simulink model "manual_model_features"  (R2020b)
settings: Solver=VariableStepAuto  StartTime=0.0  StopTime=10.0  RelTol=1e-3
undefined symbols (not defined in the file): sigbuilder_block
libraries: simulink x141
(part 1 of 3)
settings Model: Creator=99003757  LastModifiedBy=99003732
settings SFSimCC: CustomCodeUndefinedFunction=UseInterfaceOnly

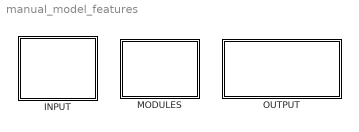
== system manual_model_features ==
  INPUT : Subsystem
  MODULES : Subsystem
  OUTPUT : Subsystem

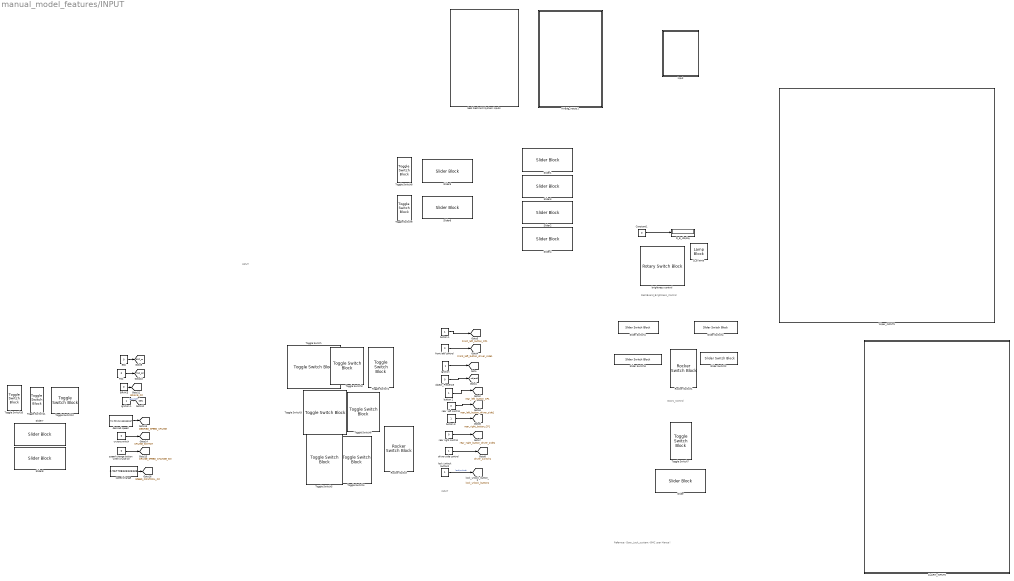
== system manual_model_features/INPUT ==
  note: INPUT
  note: INPUT
  note: DashBoard_Brightness_Control
  note: Doors_Control
  note: Refernce:-
      | Door_Lock_system:-GMC user Manua l
  ALARM_INPUTS : Subsystem
  AirBag_Inputs1 : Subsystem
  BRAKE : Constant  Value=0
  Constant1 : Constant  Value=0
  D_B lamp : LampBlock
  D_B_display : Display
  ESC : Constant  Value=0
  Input : Subsystem
  Rocker Switch : RockerSwitchBlock  LabelPosition=Bottom
      settings: Values={{'Off', 'On'}, [0 1]}
  Rocker Switch1 : RockerSwitchBlock
      settings: Values={{'Off', 'On'}, [1 0]}
  Seat Restraint System Inputs : Subsystem
  Slider{,1..8} (9 alike) : SliderBlock
  Slider Switch{1..4} (4 alike) : SliderSwitchBlock
      settings: Values={{'unlock', 'lock'}, [0 1]}
  TSC : Constant  Value=0
  Toggle Switch{,1..12} (13 alike) : ToggleSwitchBlock
  Wiper_INPUTS : Subsystem
  brightness control : RotarySwitchBlock
      settings: Values={{'Off', 'very Low', 'Low', 'medium', 'high', 'very high'}, [0 1 2 3 4 5]}
  "button 1 " : Constant
  button 2 : Constant
  button 3 : Constant
  cruise switch : Constant  Value=0
  desired speed : Constant  Value=51.90104166666667
  driver side control : Constant
  front left control : Constant  Value=0
  "ignition " : Constant
  ignition 1 : Constant
  lock /unlock button2 : Constant
  object_Presence : Constant  Value=0
  rear  left control : Constant  Value=0
  rear right control : Constant  Value=0
  speed change : Constant  Value=3.567708333333333
  "speed change button when cruise on " : Constant  Value=0
  tag scope: BRAKE_CC=global, CRUISE_SPEED_CHANGE_SW=global, CRUISE_SWITCH=global, DESIRED_SPEED_CRUISE=global, ESC_cc=global, Front_left_button_CP1=global, Front_left_button_driver_side1=global, IGN=global, SPEED_CONTROL_CC=global, TSC_CC=global, driver_switch1=global, ignition1=global, lock_unlock_button1=global, object1=global, rear_left_button_CP1=global, rear_left_button_driver_side1=global, rear_right_button_CP1=global, rear_right_button_driver_side1=global
  wires:
  object_Presence/1 -> [object1]
  driver side control/1 -> [driver_switch1]
  Constant1/1 -> D_B_display/1
  button 3/1 -> [rear_right_button_CP1]
  rear right control/1 -> [rear_right_button_driver_side1]
  "ignition "/1 -> [ignition1]
  rear  left control/1 -> [rear_left_button_driver_side1]
  lock /unlock button2/1 -> [lock_unlock_button1]  "lock/unlock"
  button 2/1 -> [rear_left_button_CP1]
  front left control/1 -> [Front_left_button_driver_side1]
  "button 1 "/1 -> [Front_left_button_CP1]
  speed change/1 -> [SPEED_CONTROL_CC]
  desired speed/1 -> [DESIRED_SPEED_CRUISE]
  ESC/1 -> [ESC_cc]
  ignition 1/1 -> [IGN]  "igswitch"
  "speed change button when cruise on "/1 -> [CRUISE_SPEED_CHANGE_SW]
  BRAKE/1 -> [BRAKE_CC]
  TSC/1 -> [TSC_CC]
  cruise switch/1 -> [CRUISE_SWITCH]

== system manual_model_features/MODULES ==
  "\tPOWER_WINDOW" : Subsystem
  ALARM_SYSTEM : Subsystem
  AirBagSystem : Subsystem
  AirBagSystem2 : Subsystem
  CRUISE_CONTROL : Subsystem
  Door_System : Subsystem
  SeatRestraintSystem1 : Subsystem
  Subsystem2 : Subsystem
  Tire Pressure Monitoring System : Subsystem
  WIPER_CONTROL : Subsystem
  system : Subsystem

== system manual_model_features/OUTPUT ==
  note: Roof light
  note: Signal status
  note: roof light
  ALARM_OUTPUT1 : Subsystem
  Air_Bag_Output : Subsystem
  Cruise_output : Subsystem
  Lamp : LampBlock
  OUTPUT : Subsystem
  OUTPUT1 : Subsystem
  OUTPUT2 : Subsystem
  Output : Subsystem
  Outputs1 : Subsystem
  TP1_Indicator : LampBlock
  TP2_Indicator : LampBlock
  TP3_Indicator : LampBlock
  TP4_Indicator : LampBlock
  automatic door lamp status : LampBlock
  delay lamp status : LampBlock

== system manual_model_features/INPUT/ALARM_INPUTS ==
  Signal Builder : Subsystem  Tag=STV Subsys  LoadFcn=sigbuilder_block('load');  StartFcn=sigbuilder_block('start');  StopFcn=sigbuilder_block('stop');  ClipboardFcn=sigbuilder_block('clipboard');  mask(Sigbuilder block){tuvar=[0:10]}
      mask help: Simulink:masks:SigbuilderBlock_MD
      mask init:
      | if ~strcmp(get_param(bdroot(gcbh),'SimulationStatus'),'stopped') tuvar = sigbuilder_block('maskInit'); end
      settings: CopyFcn=sigbuilder_block('copy');  DeleteFcn=sigbuilder_block('delete');  ModelCloseFcn=sigbuilder_block('modelClose');  PreSaveFcn=sigbuilder_block('preSave');  PauseFcn=sigbuilder_block('pause');  ContinueFcn=sigbuilder_block('continue');  NameChangeFcn=sigbuilder_block('namechange');  OpenFcn=sigbuilder_block('open',[403.5 199.2 550.5 359.55 ]);  CloseFcn=sigbuilder_block('close');
      mask Display: plot(0, 0, 100, 100,[2, 2, 32, 32, 2], [68, 8, 8, 68, 68],[32, 2], [38, 38], [32, 19, 2],[53, 60, 44], [32, 17, 17, 2],[16, 16, 31, 31]);txt = getActiveGroup(gcbh);text(2, 100, txt,'verticalAlignment', 'top');
  tag scope: AS_Doors=global, CAR_ON=global, Ignition=global, RKE=global
  wires:
  Signal Builder/1(AS_Doors) -> [AS_Doors]
  Signal Builder/2(Ignition) -> [Ignition]
  Signal Builder/3(Car_ON) -> [CAR_ON]
  Signal Builder/4(RKE) -> [RKE]

== system manual_model_features/INPUT/AirBag_Inputs1 ==
  Vehicle_Speed : RotarySwitchBlock
      settings: Values={{'50kmph', '80kmph', '100kmph', '140kmph', '180kmph', '230kmph'}, [50 80 100 140 180 230]}
  YawRateMeasure : RotarySwitchBlock
      settings: Values={{'Forward', 'Turning'}, [50 100]}

== system manual_model_features/INPUT/Input ==
  Signal Builder1 : Subsystem  Tag=STV Subsys  LoadFcn=sigbuilder_block('load');  StartFcn=sigbuilder_block('start');  StopFcn=sigbuilder_block('stop');  ClipboardFcn=sigbuilder_block('clipboard');  mask(Sigbuilder block){tuvar=[0:10]}
      mask help: Simulink:masks:SigbuilderBlock_MD
      mask init:
      | if ~strcmp(get_param(bdroot(gcbh),'SimulationStatus'),'stopped') tuvar = sigbuilder_block('maskInit'); end
      settings: CopyFcn=sigbuilder_block('copy');  DeleteFcn=sigbuilder_block('delete');  ModelCloseFcn=sigbuilder_block('modelClose');  PreSaveFcn=sigbuilder_block('preSave');  PauseFcn=sigbuilder_block('pause');  ContinueFcn=sigbuilder_block('continue');  NameChangeFcn=sigbuilder_block('namechange');  OpenFcn=sigbuilder_block('open',[6 37.5 329.25 111.75 ]);  CloseFcn=sigbuilder_block('close');
      mask Display: plot(0, 0, 100, 100,[2, 2, 32, 32, 2], [68, 8, 8, 68, 68],[32, 2], [38, 38], [32, 19, 2],[53, 60, 44], [32, 17, 17, 2],[16, 16, 31, 31]);txt = getActiveGroup(gcbh);text(2, 100, txt,'verticalAlignment', 'top');
  tag scope: ADl_Ignition_System=global, D_sys_Door1=global, D_sys_Door2=global, D_sys_Door3=global, D_sys_Door4=global, D_sys_antilock=global, accln=global
  wires:
  Signal Builder1/1(ignition status) -> [ADl_Ignition_System]
  Signal Builder1/2(Door_1) -> [D_sys_Door1]
  Signal Builder1/3(Door_2) -> [D_sys_Door2]
  Signal Builder1/4(Door_3) -> [D_sys_Door3]
  Signal Builder1/5(Door_4) -> [D_sys_Door4]
  Signal Builder1/6(antilockleature) -> [D_sys_antilock]
  Signal Builder1/7(accln) -> [accln]

== system manual_model_features/INPUT/Seat Restraint System Inputs ==
  Rotary Switch : RotarySwitchBlock
      settings: Values={{'RearAdjust', 'SeatAdjust', 'CushionAdjust', 'Lock'}, [0 1 2 3]}
  SliderForCushionAdjust : SliderBlock
  SliderForRearAdjust : SliderBlock
  SliderForSeatAdjust1 : SliderBlock
  Toggle Switch1 : ToggleSwitchBlock
      settings: Values={{'Off', 'On'}, [0 1]}
  Toggle Switch2 : ToggleSwitchBlock
      settings: Values={{'Off', 'On'}, [0 1]}
  Toggle Switch3 : ToggleSwitchBlock
      settings: Values={{'Off', 'On'}, [0 1]}

== system manual_model_features/INPUT/Wiper_INPUTS ==
  Signal Builder : Subsystem  Tag=STV Subsys  LoadFcn=sigbuilder_block('load');  StartFcn=sigbuilder_block('start');  StopFcn=sigbuilder_block('stop');  ClipboardFcn=sigbuilder_block('clipboard');  mask(Sigbuilder block){tuvar=[0:10]}
      mask help: Simulink:masks:SigbuilderBlock_MD
      mask init:
      | if ~strcmp(get_param(bdroot(gcbh),'SimulationStatus'),'stopped') tuvar = sigbuilder_block('maskInit'); end
      settings: CopyFcn=sigbuilder_block('copy');  DeleteFcn=sigbuilder_block('delete');  ModelCloseFcn=sigbuilder_block('modelClose');  PreSaveFcn=sigbuilder_block('preSave');  PauseFcn=sigbuilder_block('pause');  ContinueFcn=sigbuilder_block('continue');  NameChangeFcn=sigbuilder_block('namechange');  OpenFcn=sigbuilder_block('open',[437.6 199.2 550.4 400 ]);  CloseFcn=sigbuilder_block('close');
      mask Display: plot(0, 0, 100, 100,[2, 2, 32, 32, 2], [68, 8, 8, 68, 68],[32, 2], [38, 38], [32, 19, 2],[53, 60, 44], [32, 17, 17, 2],[16, 16, 31, 31]);txt = getActiveGroup(gcbh);text(2, 100, txt,'verticalAlignment', 'top');
  tag scope: FC_ManualInput=global, FW_Modes=global, WC_BackS=global, WC_FrontS=global, WC_Status=global
  wires:
  Signal Builder/1(FC_Modes) -> [FW_Modes]
  Signal Builder/2(FC_ManualInput) -> [FC_ManualInput]
  Signal Builder/3(WC_BackS) -> [WC_BackS]
  Signal Builder/4(WC_Fronts) -> [WC_FrontS]
  Signal Builder/5(WC_Status) -> [WC_Status]

== system manual_model_features/MODULES/	POWER_WINDOW ==
  Subsystem4 : Subsystem
  tag scope: FL_out=global, FL_warn=global, RL_out=global, RL_warn=global, RR_out=global, RR_warn=global, driver_side_output=global, driver_warn=global
  wires:
  Subsystem4/2(Out_FL) -> [FL_out]
  Subsystem4/1(Out_warn) -> [FL_warn]
  Subsystem4/4(Out_RL) -> [RL_out]
  Subsystem4/6(Out_RR) -> [RR_out]
  [object1] -> Subsystem4/2(object)
  [ignition1] -> Subsystem4/1(Ig_sw)
  Subsystem4/3(Out_RL_warn) -> [RL_warn]
  Subsystem4/8(Out_DC) -> [driver_side_output]
  Subsystem4/5(Out_RR_warn) -> [RR_warn]
  Subsystem4/7(Out_DC_warn) -> [driver_warn]

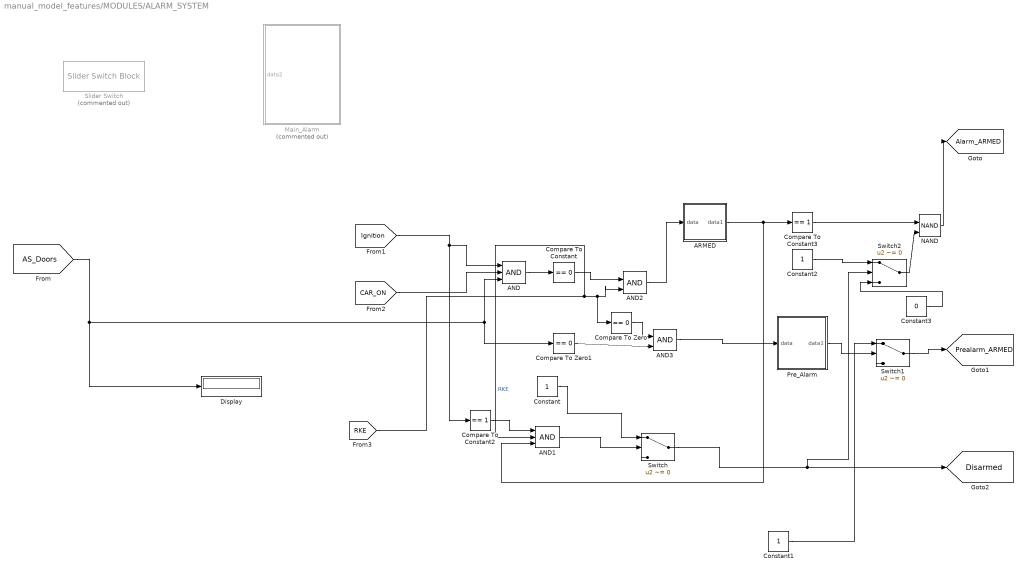
== system manual_model_features/MODULES/ALARM_SYSTEM ==
  AND : Logic  Inputs=3  IconShape=distinctive  AllPortsSameDT=off  OutDataTypeStr=boolean
  AND1 : Logic  Inputs=3  IconShape=distinctive  AllPortsSameDT=off  OutDataTypeStr=boolean
  AND2 : Logic  IconShape=distinctive  AllPortsSameDT=off  OutDataTypeStr=boolean
  AND3 : Logic  IconShape=distinctive  AllPortsSameDT=off  OutDataTypeStr=boolean
  ARMED : Stateflow chart  TreatAsAtomicUnit=on
  Compare To Constant : simulink/Logic and Bit Operations/Compare To Constant  relop===  const=0  OutDataTypeStr=boolean
  Compare To Constant2 : simulink/Logic and Bit Operations/Compare To Constant  relop===  const=1  OutDataTypeStr=boolean
  Compare To Constant3 : simulink/Logic and Bit Operations/Compare To Constant  relop===  const=1  OutDataTypeStr=boolean
  Compare To Zero : simulink/Logic and Bit Operations/Compare To Zero  relop===  OutDataTypeStr=boolean
  Compare To Zero1 : simulink/Logic and Bit Operations/Compare To Zero  relop===  OutDataTypeStr=boolean
  Constant : Constant
  Constant1 : Constant
  Constant2 : Constant
  Constant3 : Constant  Value=0
  Display : Display
  Main_Alarm : Subsystem  Commented=on
  NAND : Logic  Operator=NAND  IconShape=distinctive  AllPortsSameDT=off  OutDataTypeStr=boolean
  Pre_Alarm : Stateflow chart  TreatAsAtomicUnit=on
  Slider Switch : SliderSwitchBlock  Commented=on
      settings: Values={{'Off', 'On'}, [1 0]}
  Switch : Switch  Criteria=u2 ~= 0
  Switch1 : Switch  Criteria=u2 ~= 0
  Switch2 : Switch  Criteria=u2 ~= 0
  tag scope: Alarm_ARMED=global, Disarmed=global, Prealarm_ARMED=global
  wires:
  [RKE] -> AND1/2, Compare To Zero/1, AND2/2  "RKE"
  Constant/1 -> Switch/1
  Constant1/1 -> Switch1/1
  Compare To Zero1/1 -> AND3/2
  Compare To Constant3/1 -> NAND/1
  [CAR_ON] -> AND/2
  Compare To Zero/1 -> AND3/1
  AND2/1 -> ARMED/1(data)
  Pre_Alarm/1(data1) -> Switch1/2
  Compare To Constant/1 -> AND2/1
  AND1/1 -> Switch/2
  [Ignition] -> Compare To Constant2/1, AND/1
  AND/1 -> Compare To Constant/1
  Compare To Constant2/1 -> AND1/1
  Switch/1 -> Switch2/2, [Disarmed]
  Switch1/1 -> [Prealarm_ARMED]
  ARMED/1(data1) -> AND1/3, Compare To Constant3/1
  AND3/1 -> Pre_Alarm/1(data)
  [AS_Doors] -> Display/1, Compare To Zero1/1, AND/3
  Constant2/1 -> Switch2/1
  Switch2/1 -> NAND/2
  NAND/1 -> [Alarm_ARMED]
  Constant3/1 -> Switch2/3

== system manual_model_features/MODULES/AirBagSystem ==
  AND : Logic  IconShape=distinctive  AllPortsSameDT=off  OutDataTypeStr=boolean
  AND1 : Logic  IconShape=distinctive  AllPortsSameDT=off  OutDataTypeStr=boolean
  ActivateAirBagSensor : MATLAB Function  TreatAsAtomicUnit=on
  DetectDeceleration : Subsystem
  FrontAirBagActivation : Subsystem  TreatAsAtomicUnit=on
  Side/Front : Subsystem
  SideAirBagActivation : Subsystem  TreatAsAtomicUnit=on
  wires:
  AND/1 -> FrontAirBagActivation/1(True), FrontAirBagActivation/Enable
  Side/Front/2(In_Front1) -> AND1/1
  ActivateAirBagSensor/1(AirBagSensor) -> AND1/2, AND/2
  Side/Front/1(In_Front) -> AND/1
  AND1/1 -> SideAirBagActivation/1(True), SideAirBagActivation/Enable
  DetectDeceleration/1(Out1) -> ActivateAirBagSensor/1(SuddenDeceleration)

== system manual_model_features/MODULES/AirBagSystem2 ==
  AND : Logic  IconShape=distinctive  AllPortsSameDT=off  OutDataTypeStr=boolean
  AND1 : Logic  IconShape=distinctive  AllPortsSameDT=off  OutDataTypeStr=boolean
  ActivateAirBagSensor : MATLAB Function  TreatAsAtomicUnit=on
  DetectDeceleration : Subsystem
  FrontAirBagActivation : Subsystem  TreatAsAtomicUnit=on
  FrontAirBagActivation1 : Subsystem  TreatAsAtomicUnit=on
  Side/Front : Subsystem
  wires:
  AND/1 -> FrontAirBagActivation/1(True), FrontAirBagActivation/Enable
  AND1/1 -> FrontAirBagActivation1/1(True), FrontAirBagActivation1/Enable
  DetectDeceleration/1(Out1) -> ActivateAirBagSensor/1(SuddenDeceleration)
  ActivateAirBagSensor/1(AirBagSensor) -> AND1/2, AND/2
  Side/Front/2(In_Front1) -> AND1/1
  Side/Front/1(In_Front) -> AND/1

== system manual_model_features/MODULES/CRUISE_CONTROL ==
  note: IGN
  Display : Display
  MATLAB Function : MATLAB Function  TreatAsAtomicUnit=on
  tag scope: output_cruise=global
  wires:
  [DESIRED_SPEED_CRUISE] -> MATLAB Function/5(DESIRED_SPEED_CRUISE)
  [BRAKE_CC] -> MATLAB Function/3(BRAKE_CC)
  [CRUISE_SWITCH] -> MATLAB Function/6(cs)
  [ESC_cc] -> MATLAB Function/1(ESC_CC)
  [SPEED_CONTROL_CC] -> MATLAB Function/8(speedch)
  MATLAB Function/1(y) -> [output_cruise], Display/1  "output"
  [TSC_CC] -> MATLAB Function/2(TSC_CC)
  [IGN] -> MATLAB Function/4(IGN)
  [CRUISE_SPEED_CHANGE_SW] -> MATLAB Function/7(CRUISE_SPEED_CHANGE_SW)

== system manual_model_features/MODULES/Door_System ==
  AND : Logic  IconShape=distinctive  AllPortsSameDT=off  OutDataTypeStr=boolean
  AutomaticDoorLock : Subsystem
  Compare To Constant : simulink/Logic and Bit Operations/Compare To Constant  relop=>  const=0  OutDataTypeStr=boolean
  Display : Display
  Display1 : Display
  OR1 : Logic  Operator=OR  IconShape=distinctive  AllPortsSameDT=off  OutDataTypeStr=boolean
  delay system door lock and interior light subsystem : Subsystem
  wires:
  AutomaticDoorLock/1(Out1) -> AND/1
  AND/1 -> OR1/1, Display/1
  AutomaticDoorLock/2(Out2) -> AND/2
  Compare To Constant/1 -> OR1/2
  OR1/1 -> Display1/1
  delay system door lock and interior light subsystem/1(Out1) -> Compare To Constant/1

== system manual_model_features/MODULES/SeatRestraintSystem1 ==
  Front Seat : Subsystem  TreatAsAtomicUnit=on
  PowerLumbar : Subsystem
  Subsystem : Subsystem
  wires:
  Subsystem/2(Enable_powerSeat_Adj) -> PowerLumbar/1(PowerLumbar)
  Subsystem/1(Enable_FrontSeat_Adj) -> Front Seat/Enable, Front Seat/1(Front_Seat_Adjust)

== system manual_model_features/MODULES/Subsystem2 ==
  CloseValue : Constant  Value=0
  OpenValue : Constant  Value=100
  Subsystem : Subsystem
  Subsystem1 : Subsystem
  enabling system : Subsystem
  tag scope: output1=global, output2=global
  wires:
  enabling system/1(Outport) -> Subsystem1/1(Enable)
  enabling system/2(enableO) -> Subsystem/1(Enable)
  CloseValue/1 -> Subsystem/2(Inport)
  OpenValue/1 -> Subsystem1/2(Inport)
  Subsystem/1(Outport) -> [output2]
  Subsystem1/1(Outport) -> [output1]

== system manual_model_features/MODULES/Tire Pressure Monitoring System ==
  TP_Monitoring : Subsystem
  Tier1State : Display
  Tier2State : Display
  Tier3State : Display
  Tier4State : Display
  tierPressure1 : Constant  Value=87.46448863636364
  tierPressure2 : Constant  Value=75.64630681818181
  tierPressure3 : Constant  Value=78.37357954545455
  tierPressure4 : Constant  Value=86.10085227272727
  wires:
  TP_Monitoring/2(Out2) -> Tier2State/1
  tierPressure4/1 -> TP_Monitoring/4(tierPressure4a), TP_Monitoring/8(tierPressure4b)
  TP_Monitoring/1(Out1) -> Tier1State/1
  tierPressure1/1 -> TP_Monitoring/5(tierPressure1b), TP_Monitoring/1(tierPressure1a)
  tierPressure3/1 -> TP_Monitoring/3(tierPressure3a), TP_Monitoring/7(tierPressure3b)
  TP_Monitoring/3(Out3) -> Tier3State/1
  tierPressure2/1 -> TP_Monitoring/6(tierPressure2b), TP_Monitoring/2(tierPressure2a)
  TP_Monitoring/4(Out4) -> Tier4State/1

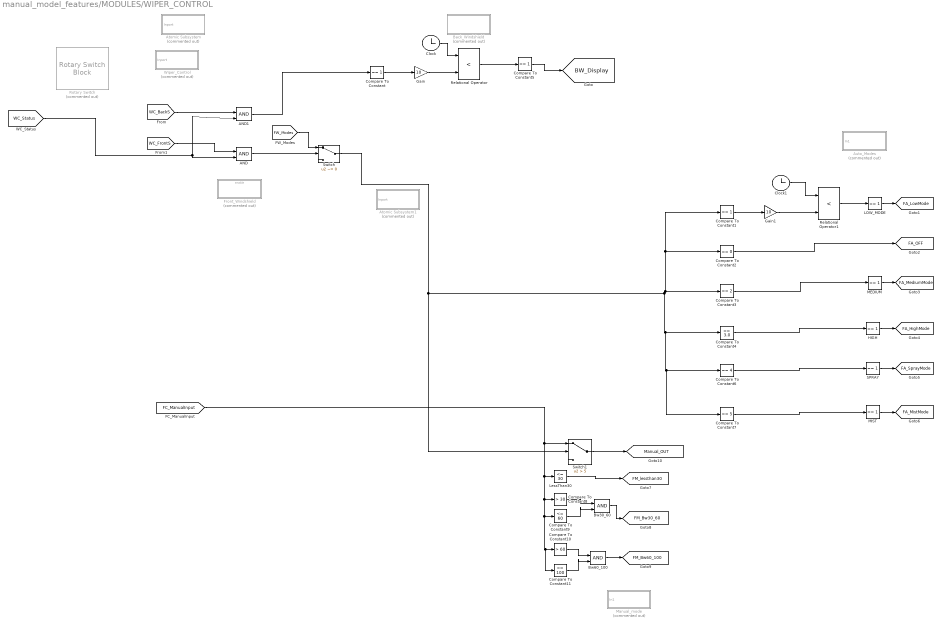
== system manual_model_features/MODULES/WIPER_CONTROL ==
  AND : Logic  IconShape=distinctive  AllPortsSameDT=off  OutDataTypeStr=boolean
  AND1 : Logic  IconShape=distinctive  AllPortsSameDT=off  OutDataTypeStr=boolean
  Atomic Subsystem : Subsystem  Commented=on  TreatAsAtomicUnit=on
  Atomic Subsystem1 : Subsystem  Commented=on  TreatAsAtomicUnit=on
  Auto_Modes : Subsystem  Commented=on
  Back_Windshield : Subsystem  Commented=on  TreatAsAtomicUnit=on
  Bw30_60 : Logic  IconShape=distinctive  AllPortsSameDT=off  OutDataTypeStr=boolean
  Bw60_100 : Logic  IconShape=distinctive  AllPortsSameDT=off  OutDataTypeStr=boolean
  Clock : Clock
      settings: Decimation=5
  Clock1 : Clock
      settings: Decimation=5
  Compare To Constant : simulink/Logic and Bit Operations/Compare To Constant  relop===  const=1  OutDataTypeStr=boolean
  Compare To Constant1 : simulink/Logic and Bit Operations/Compare To Constant  relop===  const=1  OutDataTypeStr=boolean
  Compare To Constant10 : simulink/Logic and Bit Operations/Compare To Constant  relop=>  const=60  OutDataTypeStr=boolean
  Compare To Constant11 : simulink/Logic and Bit Operations/Compare To Constant  relop=<=  const=100  OutDataTypeStr=boolean
  Compare To Constant2 : simulink/Logic and Bit Operations/Compare To Constant  relop===  const=0  OutDataTypeStr=boolean
  Compare To Constant3 : simulink/Logic and Bit Operations/Compare To Constant  relop===  const=2  OutDataTypeStr=boolean
  Compare To Constant4 : simulink/Logic and Bit Operations/Compare To Constant  relop===  const=3.0  OutDataTypeStr=boolean
  Compare To Constant5 : simulink/Logic and Bit Operations/Compare To Constant  relop===  const=1  OutDataTypeStr=boolean
  Compare To Constant6 : simulink/Logic and Bit Operations/Compare To Constant  relop===  const=4  OutDataTypeStr=boolean
  Compare To Constant7 : simulink/Logic and Bit Operations/Compare To Constant  relop===  const=5  OutDataTypeStr=boolean
  Compare To Constant8 : simulink/Logic and Bit Operations/Compare To Constant  relop=>  const=30  OutDataTypeStr=boolean
  Compare To Constant9 : simulink/Logic and Bit Operations/Compare To Constant  relop=<=  const=60  OutDataTypeStr=boolean
  Front_Windshield : Subsystem  Commented=on  TreatAsAtomicUnit=on
  Gain : Gain  Gain=10
  Gain1 : Gain  Gain=10
  HIGH : simulink/Logic and Bit Operations/Compare To Constant  relop===  const=1  OutDataTypeStr=boolean
  LOW_MODE : simulink/Logic and Bit Operations/Compare To Constant  relop===  const=1  OutDataTypeStr=boolean
  LessThan30 : simulink/Logic and Bit Operations/Compare To Constant  relop=<=  const=30  OutDataTypeStr=boolean
  MEDIUM : simulink/Logic and Bit Operations/Compare To Constant  relop===  const=1  OutDataTypeStr=boolean
  MIST : simulink/Logic and Bit Operations/Compare To Constant  relop===  const=1  OutDataTypeStr=boolean
  Manual_mode : Subsystem  Commented=on
  Relational Operator : RelationalOperator  Operator=<  OutDataTypeStr=boolean  RndMeth=Simplest
  Relational Operator1 : RelationalOperator  Operator=<  OutDataTypeStr=boolean  RndMeth=Simplest
  Rotary Switch : RotarySwitchBlock  Commented=on
      settings: Values={{'Off', 'Accessory', 'Ignition'}, [0 1 2]}
  SPRAY : simulink/Logic and Bit Operations/Compare To Constant  relop===  const=1  OutDataTypeStr=boolean
  Switch : Switch  Criteria=u2 ~= 0
  Switch1 : Switch  Criteria=u2 > Threshold  Threshold=5
  Wiper_Control : Subsystem  Commented=on  TreatAsAtomicUnit=on
  tag scope: BW_Display=global, FA_HighMode=global, FA_LowMode=global, FA_MediumMode=global, FA_MistMode=global, FA_OFF=global, FA_SprayMode=global, FM_Bw30_60=global, FM_Bw60_100=global, FM_lessthan30=global, Manual_OUT=global
  wires:
  [WC_Status] -> AND1/2, AND/2
  [WC_BackS] -> AND1/1
  [WC_FrontS] -> AND/1
  Compare To Constant/1 -> Gain/1
  Relational Operator/1 -> Compare To Constant5/1
  Compare To Constant5/1 -> [BW_Display]
  Gain/1 -> Relational Operator/2
  Clock/1 -> Relational Operator/1
  AND1/1 -> Compare To Constant/1
  AND/1 -> Switch/2
  [FW_Modes] -> Switch/1
  Compare To Constant6/1 -> SPRAY/1
  MEDIUM/1 -> [FA_MediumMode]
  HIGH/1 -> [FA_HighMode]
  LOW_MODE/1 -> [FA_LowMode]
  Relational Operator1/1 -> LOW_MODE/1
  Clock1/1 -> Relational Operator1/1
  Gain1/1 -> Relational Operator1/2
  SPRAY/1 -> [FA_SprayMode]
  MIST/1 -> [FA_MistMode]
  Compare To Constant7/1 -> MIST/1
  Compare To Constant2/1 -> [FA_OFF]
  Compare To Constant1/1 -> Gain1/1
  Switch1/1 -> [Manual_OUT]
  [FC_ManualInput] -> Compare To Constant11/1, Compare To Constant10/1, Compare To Constant9/1, Compare To Constant8/1, LessThan30/1, Switch1/1
  Compare To Constant9/1 -> Bw30_60/2
  Switch/1 -> Switch1/2, Compare To Constant7/1, Compare To Constant6/1, Compare To Constant4/1, Compare To Constant3/1, Compare To Constant1/1, Compare To Constant2/1
  LessThan30/1 -> [FM_lessthan30]
  Compare To Constant10/1 -> Bw60_100/1
  Compare To Constant8/1 -> Bw30_60/1
  Compare To Constant11/1 -> Bw60_100/2
  Bw60_100/1 -> [FM_Bw60_100]
  Bw30_60/1 -> [FM_Bw30_60]
  Compare To Constant3/1 -> MEDIUM/1
  Compare To Constant4/1 -> HIGH/1

== system manual_model_features/MODULES/system ==
  note: DOOR LOCK SYSTEM AND INTERIOR LIGHT
  note: Signal status
  note: Doors
  note: Dashboard brightness control
  note: Roof light
  Automatic_Door_lock : Subsystem
  Compare To Constant : simulink/Logic and Bit Operations/Compare To Constant  relop=>  const=0  OutDataTypeStr=boolean
  Constant1 : Constant  Value=0
  Display : Display
  Display1 : Display
  Display2 : Display
  Lamp : LampBlock
  OR1 : Logic  Operator=OR  IconShape=distinctive  AllPortsSameDT=off  OutDataTypeStr=boolean
  Rocker Switch : RockerSwitchBlock
      settings: Values={{'Off', 'On'}, [1 0]}
  Slider : SliderBlock
  Slider Switch{1..4} (4 alike) : SliderSwitchBlock
      settings: Values={{'unlock', 'lock'}, [0 1]}
  Toggle Switch : ToggleSwitchBlock
      settings: Values={{'Off', 'On'}, [0 1]}
  automatic door lamp status : LampBlock
  brightness control : RotarySwitchBlock
      settings: Values={{'Off', 'very Low', 'Low', 'medium', 'high', 'very high'}, [0 1 2 3 4 5]}
  dashboard lamp : LampBlock
  delay lamp status : LampBlock
  delay system door lock and interior light subsystem : Subsystem
  tag scope: A_D_lock=global, D_sys_lock=global
  wires:
  Constant1/1 -> Display2/1
  Compare To Constant/1 -> [D_sys_lock], OR1/2
  delay system door lock and interior light subsystem/1(Out1) -> Compare To Constant/1
  OR1/1 -> Display1/1
  Automatic_Door_lock/1(Out1) -> [A_D_lock], OR1/1, Display/1

== system manual_model_features/OUTPUT/ALARM_OUTPUT1 ==
  note: OUTPUTS
  Display : Display
  Display1 : Display
  Display2 : Display
  Lamp : LampBlock
  wires:
  [Disarmed] -> Display2/1
  [Prealarm_ARMED] -> Display1/1
  [Alarm_ARMED] -> Display/1

== system manual_model_features/OUTPUT/Air_Bag_Output ==
  note: Side Crash (Only the occupied seats are enabled with airbag deployment)
  note: Frontal Crash (Only the occupied seats are enabled with airbag deployment)
  DriverDoorUnlock : LampBlock
  DriverDoorUnlock1 : LampBlock
  DriverFront : LampBlock
  DriverFront1 : LampBlock
  FuelLock{,1..7} (8 alike) : LampBlock
  LeftDoorUnlock : LampBlock
  LeftDoorUnlock1 : LampBlock
  LeftFront : LampBlock
  LeftFront1 : LampBlock
  LeftRear : LampBlock
  LeftRear1 : LampBlock
  LeftRearDoorUnlock : LampBlock
  LeftRearDoorUnlock1 : LampBlock
  RightRear : LampBlock
  RightRear1 : LampBlock
  RightRearDoorUnlock : LampBlock
  RightRearDoorUnlock1 : LampBlock

== system manual_model_features/OUTPUT/Cruise_output ==
  Gauge : CircularGaugeBlock
  Scope : Scope
  wires:
  [output_cruise] -> Scope/1

== system manual_model_features/OUTPUT/OUTPUT ==
  Output_window_scope : Scope  NumInputPorts=4
  Warning_Scope : Scope  NumInputPorts=4
  wires:
  [RR_warn] -> Warning_Scope/3
  [RL_warn] -> Warning_Scope/2
  [FL_warn] -> Warning_Scope/1
  [FL_out] -> Output_window_scope/1
  [RL_out] -> Output_window_scope/2
  [RR_out] -> Output_window_scope/3
  [driver_side_output] -> Output_window_scope/4
  [driver_warn] -> Warning_Scope/4

== system manual_model_features/OUTPUT/OUTPUT1 ==
  Display : Display
  Display1 : Display
  wires:
  [output2] -> Display1/1
  [output1] -> Display/1

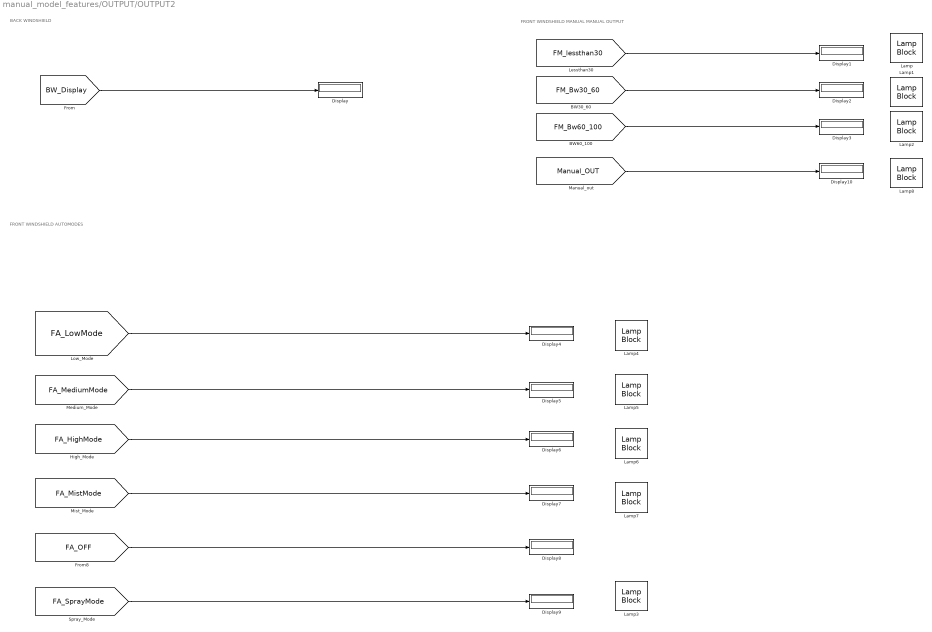
== system manual_model_features/OUTPUT/OUTPUT2 ==
  note: BACK WINDSHIELD
  note: FRONT WINDSHIELD AUTOMODES
  note: FRONT WINDSHIELD MANUAL MANUAL OUTPUT
  Display{,1..10} (11 alike) : Display
  Lamp{,1..8} (9 alike) : LampBlock
  wires:
  [BW_Display] -> Display/1
  [FM_lessthan30] -> Display1/1
  [FM_Bw30_60] -> Display2/1
  [FM_Bw60_100] -> Display3/1
  [FA_LowMode] -> Display4/1
  [FA_MediumMode] -> Display5/1
  [FA_HighMode] -> Display6/1
  [FA_MistMode] -> Display7/1
  [FA_OFF] -> Display8/1
  [FA_SprayMode] -> Display9/1
  [Manual_OUT] -> Display10/1

== system manual_model_features/OUTPUT/Output ==
  Lamp : LampBlock
  Lamp1 : LampBlock
  Lamp2 : LampBlock
  Scope3 : Scope  NumInputPorts=3
  wires:
  [D_Sys_roof] -> Scope3/1
  [A_D_lock] -> Scope3/2
  [D_sys_lock] -> Scope3/3

== system manual_model_features/OUTPUT/Outputs1 ==
  CushionAdjusted : LampBlock
  Front Seat Adjusted : LampBlock
  RearAngleOfSeatAdjust : LampBlock
  SeatUP/DownAdjusted : LampBlock

== system manual_model_features/INPUT/ALARM_INPUTS/Signal Builder ==
  Demux : Demux  Tag=STV Demux
      settings: DisplayOption=none
  FromWs : FromWorkspace  Tag=STV FromWs  VariableName=tuvar
      SigBuilderData=|
      | common.afterFinalStr = 'Extrapolate'
      | common.sampleTime = 0
      | dataSet.timeRange = [0 12]
      | dataSet.name = 'Group 1'
      | sbobj.Groups.Name = 'Group 1'
      | sbobj.Groups.Signals(1).Name = 'AS_Doors'
      | sbobj.Groups.Signals(1).XData = [0 1 2 3 4 5 6 7 8 9 10 11 12]
      | sbobj.Groups.Signals(1).YData = [0 1 1 1 1 1 1 1 1 1 1 1 1]
      | sbobj.Groups.Signals(2).Name = 'Ignition'
      | sbobj.Groups.Signals(2).XData = [0 1 2 3 4 5 6 7 8 9 10 11 12]
      | sbobj.Groups.Signals(2).YData = [0 1 1 1 1 1 1 1 1 1 1 1 1]
      | sbobj.Groups.Signals(3).Name = 'Car_ON'
      | sbobj.Groups.Signals(3).XData = [0 1 2 3 4 5 6 7 8 9 10 11 12]
      | sbobj.Groups.Signals(3).YData = [0 1 1 1 1 1 1 1 1 1 1 1 1]
      | sbobj.Groups.Signals(4).Name = 'RKE'
      | sbobj.Groups.Signals(4).XData = [0 1 2 3 4 5 6 7 8 9 10 11 12]
      | sbobj.Groups.Signals(4).YData = [0 1 1 1 1 1 2 2 2 2 2 2 2]
      | sbobj.Groups.TimeRange = [0 12]
  AS_Doors : Outport  Tag=STV Outport
  Ignition : Outport  Tag=STV Outport  Port=2
  Car_ON : Outport  Tag=STV Outport  Port=3
  RKE : Outport  Tag=STV Outport  Port=4
  wires:
  FromWs/1 -> Demux/1
  Demux/1 -> AS_Doors/1
  Demux/2 -> Ignition/1
  Demux/3 -> Car_ON/1
  Demux/4 -> RKE/1

== system manual_model_features/INPUT/Input/Signal Builder1 ==
  Demux : Demux  Tag=STV Demux  Outputs=7
      settings: DisplayOption=none
  FromWs : FromWorkspace  Tag=STV FromWs  VariableName=tuvar
      SigBuilderData=|
      | common.afterFinalStr = 'Extrapolate'
      | common.sampleTime = 0
      | dataSet.timeRange = [0 30]
      | dataSet.name = 'Group 1'
      | sbobj.Groups.Name = 'Group 1'
      | sbobj.Groups.Signals(1).Name = 'ignition status'
      | sbobj.Groups.Signals(1).XData = [0 1 2 3 4 5 6 7 8 9 10 11 12 13 14 15 16 17 18 19 20 21 22 23 24 25 26 30]
      | sbobj.Groups.Signals(1).YData = [1 1 1 1 1 0 0 0 0 0 0 1 1 1 1 1 1 1 1 1 1 0 0 0 0 0 0 0]
      | sbobj.Groups.Signals(2).Name = 'Door_1'
      | sbobj.Groups.Signals(2).XData = [0 1 2 3 4 5 6 7 8 9 10 11 12 13 14 15 16 17 18 19 20 21 22 23 24 25 26 30]
      | sbobj.Groups.Signals(2).YData = [1 1 1 1 1 1 1 1 1 1 1 1 1 1 1 1 1 1 1 1 1 0 0 0 0 0 0 0]
      | sbobj.Groups.Signals(3).Name = 'Door_2'
      | sbobj.Groups.Signals(3).XData = [0 1 2 3 4 5 6 7 8 9 10 11 12 13 14 15 16 17 18 19 20 21 22 23 24 25 26 30]
      | sbobj.Groups.Signals(3).YData = [1 1 1 1 1 1 1 1 1 1 1 1 1 1 1 1 1 1 1 1 1 0 0 0 0 0 0 0]
      | sbobj.Groups.Signals(4).Name = 'Door_3'
      | sbobj.Groups.Signals(4).XData = [0 1 2 3 4 5 6 7 8 9 10 11 12 13 14 15 16 17 18 19 20 21 22 23 24 25 26 30]
      | sbobj.Groups.Signals(4).YData = [1 1 1 1 1 1 1 1 1 1 1 1 1 1 1 1 1 1 1 1 1 0 0 0 0 0 0 0]
      | sbobj.Groups.Signals(5).Name = 'Door_4'
      | sbobj.Groups.Signals(5).XData = [0 1 2 3 4 5 6 7 8 9 10 11 12 13 14 15 16 17 18 19 20 21 22 23 24 25 26 30]
      | sbobj.Groups.Signals(5).YData = [1 1 1 1 1 1 1 1 1 1 1 1 1 1 1 1 1 1 1 1 1 0 0 0 0 0 0 0]
      | sbobj.Groups.Signals(6).Name = 'antilockleature'
      | sbobj.Groups.Signals(6).XData = [0 1 2 3 4 5 6 7 8 9 10 11 12 13 14 15 16 17 18 19 20 21 22 23 24 25 26 30]
      | sbobj.Groups.Signals(6).YData = [1 1 1 1 1 1 1 1 1 1 1 1 1 1 1 1 1 1 1 1 1 1 1 0 0 0 0 0]
      | sbobj.Groups.Signals(7).Name = 'accln'
      | sbobj.Groups.Signals(7).XData = [0 1 1 2 3 4 5 6 7 8 9 10 11 12 13 14 15 16 17 18 19 20 21 22 23 24 25 26 27 30]
      | sbobj.Groups.Signals(7).YData = [13 14 15 16 17 18 12 20 21 9 10 25 27 29 31 33 35 37 39 41 43 45 47 49 51 53 55 57 59 59]
      | sbobj.Groups.TimeRange = [0 30]
  ignition status : Outport  Tag=STV Outport
  Door_1 : Outport  Tag=STV Outport  Port=2
  Door_2 : Outport  Tag=STV Outport  Port=3
  Door_3 : Outport  Tag=STV Outport  Port=4
  Door_4 : Outport  Tag=STV Outport  Port=5
  antilockleature : Outport  Tag=STV Outport  Port=6
  accln : Outport  Tag=STV Outport  Port=7
  wires:
  FromWs/1 -> Demux/1
  Demux/1 -> ignition status/1
  Demux/2 -> Door_1/1
  Demux/3 -> Door_2/1
  Demux/4 -> Door_3/1
  Demux/5 -> Door_4/1
  Demux/6 -> antilockleature/1
  Demux/7 -> accln/1

== system manual_model_features/INPUT/Wiper_INPUTS/Signal Builder ==
  Demux : Demux  Tag=STV Demux  Outputs=5
      settings: DisplayOption=none
  FromWs : FromWorkspace  Tag=STV FromWs  VariableName=tuvar
      SigBuilderData=|
      | common.afterFinalStr = 'Extrapolate'
      | common.sampleTime = 0
      | dataSet.timeRange = [0 10]
      | dataSet.name = 'Group 1'
      | sbobj.Groups.Name = 'Group 1'
      | sbobj.Groups.Signals(1).Name = 'FC_Modes'
      | sbobj.Groups.Signals(1).XData = [0 1 2 3 4 5 6 7 8 9 10 11 12 13 14 15 16 17 18 19 20 21 22 23 24 25 26 27 28 29 30 31 32 33 34 35 36 37 38 39 40 41 42 43]
      | sbobj.Groups.Signals(1).YData = [0 1 1 1 1 1 1 1 1 1 1 1 2 2 2 2 2 2 2 2 3 3 3 3 3 4 4 4 4 4 5 5 5 6 6 6 6 6 6 6 6 6 6 6]
      | sbobj.Groups.Signals(2).Name = 'FC_ManualInput'
      | sbobj.Groups.Signals(2).XData = [0 1 2 3 4 5 6 7 8 9 10 11 12 13 14 15 16 17 18 19 20 21 22 23 24 25 26 27 28 29 30 31 32 33 34 35 36 37 38 39 40 41 42 43]
      | sbobj.Groups.Signals(2).YData = [0 0 0 0 0 0 0 0 0 0 0 0 0 0 0 0 0 0 0 0 0 0 0 0 0 0 0 0 0 0 0 0 0 0 15 20 36 50 65 69 80 85 90 98]
      | sbobj.Groups.Signals(3).Name = 'WC_BackS'
      | sbobj.Groups.Signals(3).XData = [0 1 2 3 4 5 6 7 8 9 10 11 12 13 14 15 16 17 18 19 20 21 22 23 24 25 26 27 28 29 30 31 32 33 34 35 36 37 38 39 40 41 42 43]
      | sbobj.Groups.Signals(3).YData = [0 1 1 1 1 1 1 1 1 1 1 1 0 0 0 0 0 0 0 0 0 0 0 0 0 0 0 0 0 0 0 0 0 0 0 0 0 0 0 0 0 0 0 0]
      | sbobj.Groups.Signals(4).Name = 'WC_Fronts'
      | sbobj.Groups.Signals(4).XData = [0 1 2 3 4 5 6 7 8 9 10 11 12 13 14 15 16 17 18 19 20 21 22 23 24 25 26 27 28 29 30 31 32 33 34 35 36 37 38 39 40 41 42 43]
      | sbobj.Groups.Signals(4).YData = [0 1 1 1 1 1 1 1 1 1 1 1 1 1 1 1 1 1 1 1 1 1 1 1 1 1 1 1 1 1 1 1 1 1 1 1 1 1 1 1 1 1 1 1]
      | sbobj.Groups.Signals(5).Name = 'WC_Status'
      | sbobj.Groups.Signals(5).XData = [0 1 2 3 4 5 6 7 8 9 10 11 12 13 14 15 16 17 18 19 20 21 22 23 24 25 26 27 28 29 30 31 32 33 34 35 36 37 38 39 40 41 42 43]
      | sbobj.Groups.Signals(5).YData = [0 1 1 1 1 1 1 1 1 1 1 1 1 1 1 1 1 1 1 1 1 1 1 1 1 1 1 1 1 1 1 1 1 1 1 1 1 1 1 1 1 1 1 1]
  FC_Modes : Outport  Tag=STV Outport
  FC_ManualInput : Outport  Tag=STV Outport  Port=2
  WC_BackS : Outport  Tag=STV Outport  Port=3
  WC_Fronts : Outport  Tag=STV Outport  Port=4
  WC_Status : Outport  Tag=STV Outport  Port=5
  wires:
  FromWs/1 -> Demux/1
  Demux/1 -> FC_Modes/1
  Demux/2 -> FC_ManualInput/1
  Demux/3 -> WC_BackS/1
  Demux/4 -> WC_Fronts/1
  Demux/5 -> WC_Status/1

== system manual_model_features/MODULES/	POWER_WINDOW/Subsystem4 ==
  Ig_sw : Inport
  object : Inport  Port=2
  Front_left_subsystem : Subsystem
  Rear_right_Subsystem : Subsystem
  driver_control_Subsystem : Subsystem
  rear_left_Subsystem : Subsystem
  Out_warn : Outport
  Out_FL : Outport  Port=2
  Out_RL_warn : Outport  Port=3
  Out_RL : Outport  Port=4
  Out_RR_warn : Outport  Port=5
  Out_RR : Outport  Port=6
  Out_DC_warn : Outport  Port=7
  Out_DC : Outport  Port=8
  wires:
  [lock_unlock_button1] -> Front_left_subsystem/1(lock/unlock), Rear_right_Subsystem/1(lock/unlock), rear_left_Subsystem/1(lock/unlock)  "lock/unlock"
  Ig_sw/1 -> Rear_right_Subsystem/Enable, rear_left_Subsystem/Enable, driver_control_Subsystem/Enable, Front_left_subsystem/Enable
  object/1 -> Front_left_subsystem/4(object), driver_control_Subsystem/2(object), Rear_right_Subsystem/4(object), rear_left_Subsystem/4(object)  "object"
  Front_left_subsystem/2(Outport1) -> Out_FL/1
  Front_left_subsystem/1(Outport) -> Out_warn/1
  rear_left_Subsystem/2(Outport1) -> Out_RL/1
  rear_left_Subsystem/1(Outport) -> Out_RL_warn/1
  Rear_right_Subsystem/2(Outport1) -> Out_RR/1
  Rear_right_Subsystem/1(Outport) -> Out_RR_warn/1
  driver_control_Subsystem/2(Outport1) -> Out_DC/1
  driver_control_Subsystem/1(Outport) -> Out_DC_warn/1
  [Front_left_button_CP1] -> Front_left_subsystem/2(In_fl_b)
  [Front_left_button_driver_side1] -> Front_left_subsystem/3(In_fl_Dc)
  [rear_left_button_CP1] -> rear_left_Subsystem/2(In2)
  [rear_left_button_driver_side1] -> rear_left_Subsystem/3(In3)
  [rear_right_button_CP1] -> Rear_right_Subsystem/2(In2)
  [rear_right_button_driver_side1] -> Rear_right_Subsystem/3(In3)
  [driver_switch1] -> driver_control_Subsystem/1(In1)

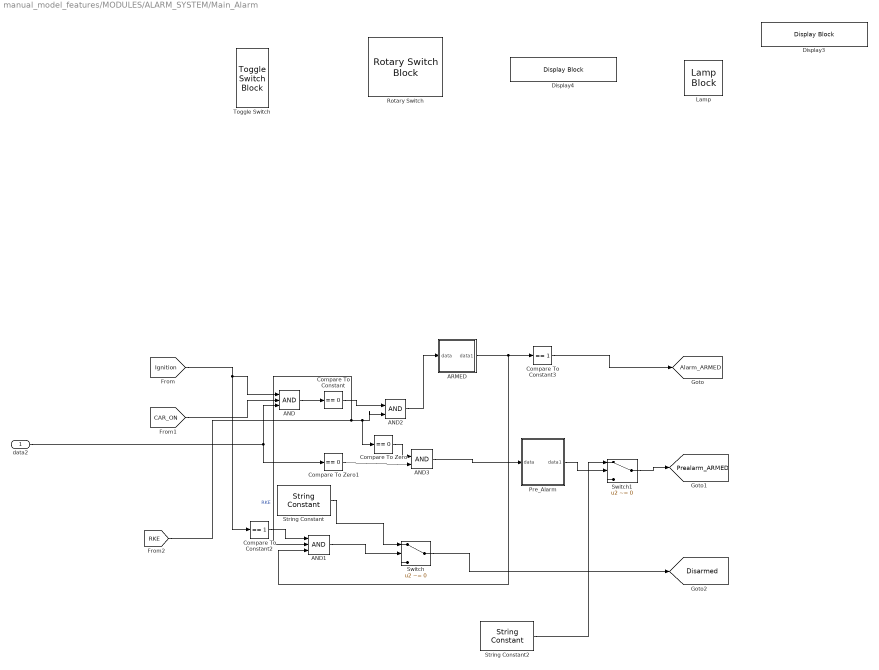
== system manual_model_features/MODULES/ALARM_SYSTEM/Main_Alarm ==
  data2 : Inport
  AND : Logic  Inputs=3  IconShape=distinctive  AllPortsSameDT=off  OutDataTypeStr=boolean
  AND1 : Logic  Inputs=3  IconShape=distinctive  AllPortsSameDT=off  OutDataTypeStr=boolean
  AND2 : Logic  IconShape=distinctive  AllPortsSameDT=off  OutDataTypeStr=boolean
  AND3 : Logic  IconShape=distinctive  AllPortsSameDT=off  OutDataTypeStr=boolean
  ARMED : Stateflow chart  TreatAsAtomicUnit=on
  Compare To Constant : simulink/Logic and Bit Operations/Compare To Constant  relop===  const=0  OutDataTypeStr=boolean
  Compare To Constant2 : simulink/Logic and Bit Operations/Compare To Constant  relop===  const=1  OutDataTypeStr=boolean
  Compare To Constant3 : simulink/Logic and Bit Operations/Compare To Constant  relop===  const=1  OutDataTypeStr=boolean
  Compare To Zero : simulink/Logic and Bit Operations/Compare To Zero  relop===  OutDataTypeStr=boolean
  Compare To Zero1 : simulink/Logic and Bit Operations/Compare To Zero  relop===  OutDataTypeStr=boolean
  Display3 : DisplayBlock  LabelPosition=Hide  Format=short  Transparency=1
  Display4 : DisplayBlock  LabelPosition=Hide  Format=short  Transparency=1
  Lamp : LampBlock
  Pre_Alarm : Stateflow chart  TreatAsAtomicUnit=on
  Rotary Switch : RotarySwitchBlock
      settings: Values={{'zero', 'one', 'Unlocking'}, [0 1 2]}
  String Constant : StringConstant  String="\"DISARMED!\""
  String Constant2 : StringConstant  String="\"Horn And Lights are ON!\""
  Switch : Switch  Criteria=u2 ~= 0
  Switch1 : Switch  Criteria=u2 ~= 0
  Toggle Switch : ToggleSwitchBlock
      settings: Values={{'Off', 'On'}, [0 1]}
  tag scope: Alarm_ARMED=global, Disarmed=global, Prealarm_ARMED=global
  wires:
  [Ignition] -> Compare To Constant2/1, AND/1
  AND/1 -> Compare To Constant/1
  [CAR_ON] -> AND/2
  ARMED/1(data1) -> AND1/3, Compare To Constant3/1
  data2/1 -> Compare To Zero1/1, AND/3
  Compare To Constant2/1 -> AND1/1
  [RKE] -> AND1/2, Compare To Zero/1, AND2/2  "RKE"
  AND1/1 -> Switch/2
  String Constant/1 -> Switch/1
  Switch/1 -> [Disarmed]
  Pre_Alarm/1(data1) -> Switch1/2
  String Constant2/1 -> Switch1/1
  Compare To Constant/1 -> AND2/1
  Compare To Constant3/1 -> [Alarm_ARMED]
  AND2/1 -> ARMED/1(data)
  Compare To Zero/1 -> AND3/1
  AND3/1 -> Pre_Alarm/1(data)
  Compare To Zero1/1 -> AND3/2
  Switch1/1 -> [Prealarm_ARMED]

== system manual_model_features/MODULES/AirBagSystem/DetectDeceleration ==
  ConstantVehicleSpeed : Constant  Value=50
  DetectDeceleration : Sum  Inputs=+-
  SuddenDeceleration : RelationalOperator  OutDataTypeStr=boolean  RndMeth=Simplest
  Value : Constant  Value=60
  Out1 : Outport
  wires:
  DetectDeceleration/1 -> SuddenDeceleration/1
  Value/1 -> SuddenDeceleration/2
  SuddenDeceleration/1 -> Out1/1
  [VehicleSpeed] -> DetectDeceleration/1
  ConstantVehicleSpeed/1 -> DetectDeceleration/2

== system manual_model_features/MODULES/AirBagSystem/FrontAirBagActivation ==
  True : Inport
  Enable : EnablePort
  Compare To Constant{,1..3} (4 alike) : simulink/Logic and Bit Operations/Compare To Constant  relop===  const=1  OutDataTypeStr=boolean
  DriverFrontAirBagActive : Subsystem  TreatAsAtomicUnit=on
  LeftFrontAirBagActive : Subsystem  TreatAsAtomicUnit=on
  LeftRearAirBagActive : Subsystem  TreatAsAtomicUnit=on
  RightRearAirBagActive : Subsystem  TreatAsAtomicUnit=on
  Switch{,1..3} (4 alike) : Switch  Criteria=u2 > Threshold
  WeightSensor : MATLAB Function  TreatAsAtomicUnit=on
  wires:
  WeightSensor/2(L_FRONT) -> Compare To Constant1/1
  [L_Front] -> WeightSensor/2(l_front)
  [Driver] -> WeightSensor/1(driver)
  WeightSensor/1(DRIVER) -> Compare To Constant/1
  WeightSensor/3(L_REAR) -> Compare To Constant2/1
  WeightSensor/4(R_REAR) -> Compare To Constant3/1
  [R_Rear] -> WeightSensor/4(r_rear)
  [L_Rear] -> WeightSensor/3(l_rear)
  True/1 -> Switch3/2, Switch2/2, Switch1/2, Switch/2
  Compare To Constant/1 -> Switch/1
  Switch/1 -> DriverFrontAirBagActive/Trigger, DriverFrontAirBagActive/1(In1)
  Compare To Constant1/1 -> Switch1/1
  Switch1/1 -> LeftFrontAirBagActive/1(In2), LeftFrontAirBagActive/Trigger
  Compare To Constant2/1 -> Switch2/1
  Switch2/1 -> LeftRearAirBagActive/Trigger, LeftRearAirBagActive/1(In1)
  Compare To Constant3/1 -> Switch3/1
  Switch3/1 -> RightRearAirBagActive/1(In2), RightRearAirBagActive/Trigger

== system manual_model_features/MODULES/AirBagSystem/Side//Front ==
  CheckYawRateForFront : RelationalOperator  Operator===  OutDataTypeStr=boolean  RndMeth=Simplest
  CheckYawRateForSide : RelationalOperator  Operator===  OutDataTypeStr=boolean  RndMeth=Simplest
  Val_Front : Constant  Value=50
  Val_Side : Constant  Value=100
  In_Front : Outport
  In_Front1 : Outport  Port=2
  wires:
  Val_Front/1 -> CheckYawRateForFront/2
  [YawRate] -> CheckYawRateForSide/1, CheckYawRateForFront/1
  CheckYawRateForFront/1 -> In_Front/1
  Val_Side/1 -> CheckYawRateForSide/2
  CheckYawRateForSide/1 -> In_Front1/1

== system manual_model_features/MODULES/AirBagSystem/SideAirBagActivation ==
  True : Inport
  Enable : EnablePort
  Compare To Constant{,1..3} (4 alike) : simulink/Logic and Bit Operations/Compare To Constant  relop===  const=1  OutDataTypeStr=boolean
  DriverSideAirBagActive : Subsystem  TreatAsAtomicUnit=on
  LeftFronrSeatAirBagActive : Subsystem  TreatAsAtomicUnit=on
  LeftRearAirBagActive : Subsystem  TreatAsAtomicUnit=on
  RightRearAirBagActive : Subsystem  TreatAsAtomicUnit=on
  Switch{,1..3} (4 alike) : Switch  Criteria=u2 > Threshold
  WeightSensor : MATLAB Function  TreatAsAtomicUnit=on
  wires:
  Switch2/1 -> LeftRearAirBagActive/Trigger, LeftRearAirBagActive/1(In1)
  WeightSensor/2(L_FRONT) -> Compare To Constant1/1
  WeightSensor/3(L_REAR) -> Compare To Constant2/1
  WeightSensor/4(R_REAR) -> Compare To Constant3/1
  [L_Front] -> WeightSensor/2(l_front)
  Compare To Constant1/1 -> Switch1/1
  [R_Rear] -> WeightSensor/4(r_rear)
  True/1 -> Switch3/2, Switch2/2, Switch1/2, Switch/2
  Switch/1 -> DriverSideAirBagActive/Trigger, DriverSideAirBagActive/1(In1)
  [Driver] -> WeightSensor/1(driver)
  Switch1/1 -> LeftFronrSeatAirBagActive/1(In2), LeftFronrSeatAirBagActive/Trigger
  [L_Rear] -> WeightSensor/3(l_rear)
  WeightSensor/1(DRIVER) -> Compare To Constant/1
  Compare To Constant3/1 -> Switch3/1
  Compare To Constant2/1 -> Switch2/1
  Compare To Constant/1 -> Switch/1
  Switch3/1 -> RightRearAirBagActive/1(In2), RightRearAirBagActive/Trigger

== system manual_model_features/MODULES/AirBagSystem2/DetectDeceleration ==
  ConstantVehicleSpeed : Constant  Value=50
  DetectDeceleration : Sum  Inputs=+-
  SuddenDeceleration : RelationalOperator  OutDataTypeStr=boolean  RndMeth=Simplest
  Value : Constant  Value=60
  VehicleSpeed : Constant  Value=180
  Out1 : Outport
  wires:
  DetectDeceleration/1 -> SuddenDeceleration/1
  Value/1 -> SuddenDeceleration/2
  SuddenDeceleration/1 -> Out1/1
  VehicleSpeed/1 -> DetectDeceleration/1
  ConstantVehicleSpeed/1 -> DetectDeceleration/2

== system manual_model_features/MODULES/AirBagSystem2/FrontAirBagActivation ==
  True : Inport
  Enable : EnablePort
  Compare To Constant{,1..3} (4 alike) : simulink/Logic and Bit Operations/Compare To Constant  relop===  const=1  OutDataTypeStr=boolean
  Driver : Constant
  DriverFrontAirBagActive : Subsystem  TreatAsAtomicUnit=on
  L_Front : Constant
  L_Rear : Constant
  LeftFrontAirBagActive : Subsystem  TreatAsAtomicUnit=on
  LeftRearAirBagActive : Subsystem  TreatAsAtomicUnit=on
  R_Rear : Constant  Value=0
  RightRearAirBagActive : Subsystem  TreatAsAtomicUnit=on
  Switch{,1..3} (4 alike) : Switch  Criteria=u2 > Threshold
  WeightSensor : MATLAB Function  TreatAsAtomicUnit=on
  wires:
  WeightSensor/2(L_FRONT) -> Compare To Constant1/1
  L_Front/1 -> WeightSensor/2(l_front)
  Driver/1 -> WeightSensor/1(driver)
  WeightSensor/1(DRIVER) -> Compare To Constant/1
  WeightSensor/3(L_REAR) -> Compare To Constant2/1
  WeightSensor/4(R_REAR) -> Compare To Constant3/1
  R_Rear/1 -> WeightSensor/4(r_rear)
  L_Rear/1 -> WeightSensor/3(l_rear)
  True/1 -> Switch3/2, Switch2/2, Switch1/2, Switch/2
  Compare To Constant/1 -> Switch/1
  Switch/1 -> DriverFrontAirBagActive/Trigger, DriverFrontAirBagActive/1(In1)
  Compare To Constant1/1 -> Switch1/1
  Switch1/1 -> LeftFrontAirBagActive/1(In2), LeftFrontAirBagActive/Trigger
  Compare To Constant2/1 -> Switch2/1
  Switch2/1 -> LeftRearAirBagActive/Trigger, LeftRearAirBagActive/1(In1)
  Compare To Constant3/1 -> Switch3/1
  Switch3/1 -> RightRearAirBagActive/1(In2), RightRearAirBagActive/Trigger

== system manual_model_features/MODULES/AirBagSystem2/FrontAirBagActivation1 ==
  True : Inport
  Enable : EnablePort
  Compare To Constant{,1..3} (4 alike) : simulink/Logic and Bit Operations/Compare To Constant  relop===  const=1  OutDataTypeStr=boolean
  Driver : Constant
  DriverSideAirBagActive : Subsystem  TreatAsAtomicUnit=on
  L_Front : Constant
  L_Rear : Constant  Value=0
  LeftFronrSeatAirBagActive : Subsystem  TreatAsAtomicUnit=on
  LeftRearAirBagActive : Subsystem  TreatAsAtomicUnit=on
  R_Rear : Constant
  RightRearAirBagActive : Subsystem  TreatAsAtomicUnit=on
  Switch{,1..3} (4 alike) : Switch  Criteria=u2 > Threshold
  WeightSensor : MATLAB Function  TreatAsAtomicUnit=on
  wires:
  Switch2/1 -> LeftRearAirBagActive/Trigger, LeftRearAirBagActive/1(In1)
  WeightSensor/2(L_FRONT) -> Compare To Constant1/1
  WeightSensor/3(L_REAR) -> Compare To Constant2/1
  WeightSensor/4(R_REAR) -> Compare To Constant3/1
  L_Front/1 -> WeightSensor/2(l_front)
  Compare To Constant1/1 -> Switch1/1
  R_Rear/1 -> WeightSensor/4(r_rear)
  True/1 -> Switch3/2, Switch2/2, Switch1/2, Switch/2
  Switch/1 -> DriverSideAirBagActive/Trigger, DriverSideAirBagActive/1(In1)
  Driver/1 -> WeightSensor/1(driver)
  Switch1/1 -> LeftFronrSeatAirBagActive/1(In2), LeftFronrSeatAirBagActive/Trigger
  L_Rear/1 -> WeightSensor/3(l_rear)
  WeightSensor/1(DRIVER) -> Compare To Constant/1
  Compare To Constant3/1 -> Switch3/1
  Compare To Constant2/1 -> Switch2/1
  Compare To Constant/1 -> Switch/1
  Switch3/1 -> RightRearAirBagActive/1(In2), RightRearAirBagActive/Trigger

== system manual_model_features/MODULES/AirBagSystem2/Side//Front ==
  CheckYawRateForFront : RelationalOperator  Operator===  OutDataTypeStr=boolean  RndMeth=Simplest
  CheckYawRateForSide : RelationalOperator  Operator===  OutDataTypeStr=boolean  RndMeth=Simplest
  Val_Front : Constant  Value=50
  Val_Side : Constant  Value=100
  YawRate : Constant  Value=100
  In_Front : Outport
  In_Front1 : Outport  Port=2
  wires:
  Val_Front/1 -> CheckYawRateForFront/2
  YawRate/1 -> CheckYawRateForSide/1, CheckYawRateForFront/1
  CheckYawRateForFront/1 -> In_Front/1
  Val_Side/1 -> CheckYawRateForSide/2
  CheckYawRateForSide/1 -> In_Front1/1

== system manual_model_features/MODULES/Door_System/AutomaticDoorLock ==
  A_D_accln : Constant  Value=15.43496621621622
  A_D_ignition : Constant
  Constant : Constant
  If : If  IfExpression=u1>=13  ElseIfExpressions=u1<13  ShowElse=off
  If Action Subsystem : Subsystem  TreatAsAtomicUnit=on
  If Action Subsystem1 : Subsystem  TreatAsAtomicUnit=on
  OR : Logic  Operator=OR  IconShape=distinctive  AllPortsSameDT=off  OutDataTypeStr=boolean
  reset : Constant  Value=0
  Out1 : Outport
  Out2 : Outport  Port=2
  wires:
  Constant/1 -> If Action Subsystem/1(In1)
  If Action Subsystem/1(Out1) -> OR/1
  If/1 -> If Action Subsystem/Action
  If/2 -> If Action Subsystem1/Action
  If Action Subsystem1/1(Out1) -> OR/2
  A_D_ignition/1 -> Out1/1
  OR/1 -> Out2/1
  A_D_accln/1 -> If/1
  reset/1 -> If Action Subsystem1/1(In1)

== system manual_model_features/MODULES/Door_System/delay system door lock and interior light subsystem ==
  note: D_s ys_Door3
  note: D_sys_Door2
  note: ys_Door4
  AND : Logic  Inputs=5  IconShape=distinctive  AllPortsSameDT=off  OutDataTypeStr=boolean
  Add : Sum
  Antilockfeature : Constant
  Compare To Constant : simulink/Logic and Bit Operations/Compare To Constant  relop===  const=0  OutDataTypeStr=boolean
  Constant4 : Constant  Value=0
  Constant5 : Constant  Value=0
  D_Sys_Door1 : Constant
  D_sys_Door2 : Constant
  D_sys_Door4 : Constant
  D_sys_roof : Logic  Inputs=4  IconShape=distinctive  AllPortsSameDT=off  OutDataTypeStr=boolean
  Data Type Conversion : DataTypeConversion
  Delay1 : Delay  DelayLength=1
  Display : Display
  Display1 : Display
  Repeating Sequence Stair : simulink/Sources/Repeating Sequence Stair  OutValues=[1 1]  tsamp=-1  OutMin=[]  OutMax=[]  OutDataTypeStr=double  OutputDataTypeScalingMode=double  OutDataType=fixdt(0,8)  ConRadixGroup=Best Precision: Vector-wise  OutScaling=2^-12
  Scope : Scope
  Switch : Switch  Threshold=5
  Switch1 : Switch
  ys_Door3 : Constant
  Out1 : Outport
  wires:
  Switch1/1 -> Scope/1, Out1/1, Delay1/1, Display/1
  Antilockfeature/1 -> AND/5
  Repeating Sequence Stair/1 -> Switch1/2
  Delay1/1 -> Add/2
  Constant5/1 -> Switch1/3
  Constant4/1 -> Switch/1
  Add/1 -> Switch/2, Switch/3
  Switch/1 -> Switch1/1
  AND/1 -> Data Type Conversion/1
  ys_Door3/1 -> D_sys_roof/3, AND/3
  D_sys_Door4/1 -> D_sys_roof/4, AND/4
  D_sys_roof/1 -> Compare To Constant/1
  D_Sys_Door1/1 -> D_sys_roof/1, AND/1
  D_sys_Door2/1 -> D_sys_roof/2, AND/2
  Compare To Constant/1 -> Display1/1
  Data Type Conversion/1 -> Add/1

== system manual_model_features/MODULES/SeatRestraintSystem1/Front Seat ==
  Front_Seat_Adjust : Inport
  Enable : EnablePort
  Adjust seat angle1 : Constant  Value=79.6256188118812
  Compare To Constant : simulink/Logic and Bit Operations/Compare To Constant  relop=>  const=0  OutDataTypeStr=boolean
  Enable Adjustment mode1 : Switch  Criteria=u2 > Threshold
  Slider to set the position of seat1 : SliderBlock
  "adjustment : Front / Back1" : Display
  wires:
  Adjust seat angle1/1 -> Enable Adjustment mode1/1
  Front_Seat_Adjust/1 -> Enable Adjustment mode1/2
  Enable Adjustment mode1/1 -> Compare To Constant/1
  Compare To Constant/1 -> "adjustment : Front / Back1"/1

== system manual_model_features/MODULES/SeatRestraintSystem1/PowerLumbar ==
  PowerLumbar : Inport
  PowerSeat : Subsystem  TreatAsAtomicUnit=on
  wires:
  PowerLumbar/1 -> PowerSeat/3(CushionAdjust), PowerSeat/2(SeatAdjust), PowerSeat/1(RearAdjust), PowerSeat/Enable

== system manual_model_features/MODULES/SeatRestraintSystem1/Subsystem ==
  AND : Logic  IconShape=distinctive  AllPortsSameDT=off  OutDataTypeStr=boolean
  AND1 : Logic  IconShape=distinctive  AllPortsSameDT=off  OutDataTypeStr=boolean
  FrontSeat : Constant
  HandleOn : Constant
  Power Seat : Constant
  Enable_FrontSeat_Adj : Outport
  Enable_powerSeat_Adj : Outport  Port=2
  wires:
  AND/1 -> Enable_FrontSeat_Adj/1
  Power Seat/1 -> AND1/2
  HandleOn/1 -> AND1/1, AND/1
  FrontSeat/1 -> AND/2
  AND1/1 -> Enable_powerSeat_Adj/1

== system manual_model_features/MODULES/Subsystem2/Subsystem ==
  Enable : Inport
  Inport : Inport  Port=2
  Enabled Subsystem : Subsystem  TreatAsAtomicUnit=on
  Outport : Outport
  wires:
  Enabled Subsystem/1(Outport) -> Outport/1
  Inport/1 -> Enabled Subsystem/1(In1)
  Enable/1 -> Enabled Subsystem/Enable

== system manual_model_features/MODULES/Subsystem2/Subsystem1 ==
  Enable : Inport
  Inport : Inport  Port=2
  Enabled Subsystem1 : Subsystem  TreatAsAtomicUnit=on
  Outport : Outport
  wires:
  Inport/1 -> Enabled Subsystem1/1(In1)
  Enabled Subsystem1/1(Outport) -> Outport/1
  Enable/1 -> Enabled Subsystem1/Enable

== system manual_model_features/MODULES/Subsystem2/enabling system ==
  Chart : Stateflow chart  TreatAsAtomicUnit=on
  Close : Constant
  Open : Constant  Value=0
  Outport : Outport
  enableO : Outport  Port=2
  wires:
  Chart/1(enableC) -> Outport/1
  Close/1 -> Chart/1(closeButton)
  Chart/2(enableO) -> enableO/1
  Open/1 -> Chart/2(openButton)

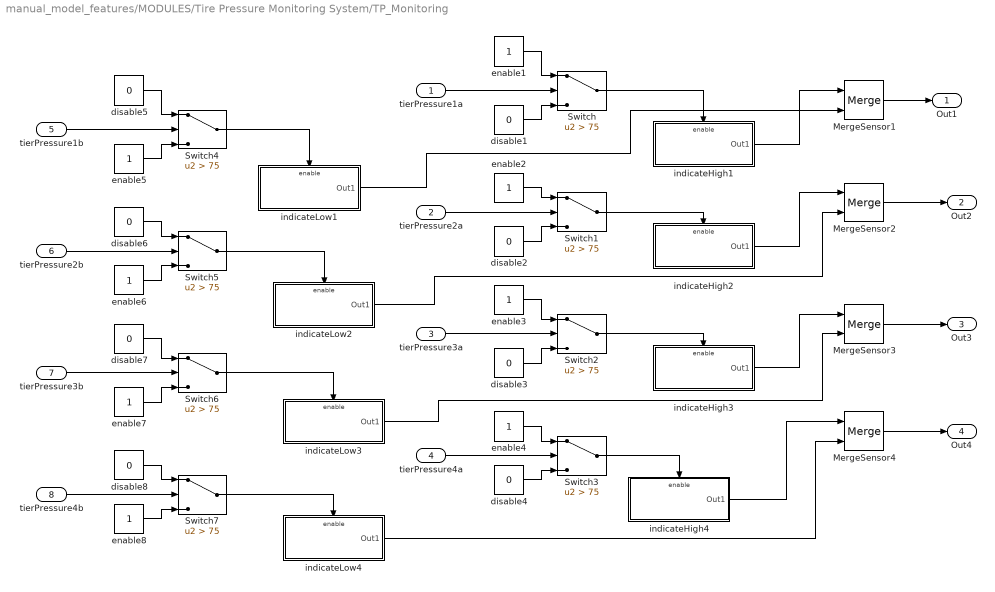
== system manual_model_features/MODULES/Tire Pressure Monitoring System/TP_Monitoring ==
  tierPressure1a : Inport
  tierPressure2a : Inport  Port=2
  tierPressure3a : Inport  Port=3
  tierPressure4a : Inport  Port=4
  tierPressure1b : Inport  Port=5
  tierPressure2b : Inport  Port=6
  tierPressure3b : Inport  Port=7
  tierPressure4b : Inport  Port=8
  MergeSensor{1..4} (4 alike) : Merge
  Switch{,1..7} (8 alike) : Switch  Criteria=u2 > Threshold  Threshold=75
  disable{1..8} (8 alike) : Constant  Value=0
  enable{1..8} (8 alike) : Constant
  indicateHigh1 : Subsystem  TreatAsAtomicUnit=on
  indicateHigh2 : Subsystem  TreatAsAtomicUnit=on
  indicateHigh3 : Subsystem  TreatAsAtomicUnit=on
  indicateHigh4 : Subsystem  TreatAsAtomicUnit=on
  indicateLow1 : Subsystem  TreatAsAtomicUnit=on
  indicateLow2 : Subsystem  TreatAsAtomicUnit=on
  indicateLow3 : Subsystem  TreatAsAtomicUnit=on
  indicateLow4 : Subsystem  TreatAsAtomicUnit=on
  Out1 : Outport
  Out2 : Outport  Port=2
  Out3 : Outport  Port=3
  Out4 : Outport  Port=4
  wires:
  enable1/1 -> Switch/1
  tierPressure3a/1 -> Switch2/2
  disable1/1 -> Switch/3
  disable3/1 -> Switch2/3
  enable2/1 -> Switch1/1
  tierPressure1a/1 -> Switch/2
  disable4/1 -> Switch3/3
  disable2/1 -> Switch1/3
  enable4/1 -> Switch3/1
  tierPressure2a/1 -> Switch1/2
  tierPressure4a/1 -> Switch3/2
  enable3/1 -> Switch2/1
  disable8/1 -> Switch7/1
  enable8/1 -> Switch7/3
  disable6/1 -> Switch5/1
  enable6/1 -> Switch5/3
  enable7/1 -> Switch6/3
  enable5/1 -> Switch4/3
  disable5/1 -> Switch4/1
  tierPressure2b/1 -> Switch5/2
  tierPressure3b/1 -> Switch6/2
  tierPressure1b/1 -> Switch4/2
  disable7/1 -> Switch6/1
  tierPressure4b/1 -> Switch7/2
  MergeSensor1/1 -> Out1/1
  MergeSensor2/1 -> Out2/1
  MergeSensor3/1 -> Out3/1
  MergeSensor4/1 -> Out4/1
  Switch3/1 -> indicateHigh4/Enable
  Switch2/1 -> indicateHigh3/Enable
  Switch1/1 -> indicateHigh2/Enable
  Switch/1 -> indicateHigh1/Enable
  Switch7/1 -> indicateLow4/Enable
  Switch6/1 -> indicateLow3/Enable
  Switch5/1 -> indicateLow2/Enable
  Switch4/1 -> indicateLow1/Enable
  indicateHigh1/1(Out1) -> MergeSensor1/1
  indicateLow1/1(Out1) -> MergeSensor1/2
  indicateHigh2/1(Out1) -> MergeSensor2/1
  indicateLow2/1(Out1) -> MergeSensor2/2
  indicateHigh3/1(Out1) -> MergeSensor3/1
  indicateLow3/1(Out1) -> MergeSensor3/2
  indicateHigh4/1(Out1) -> MergeSensor4/1
  indicateLow4/1(Out1) -> MergeSensor4/2

== system manual_model_features/MODULES/WIPER_CONTROL/Atomic Subsystem ==
  Inport : Inport
  Clock : Clock
      settings: Decimation=5
  Compare To Constant : simulink/Logic and Bit Operations/Compare To Constant  relop===  const=1  OutDataTypeStr=boolean
  Compare To Constant5 : simulink/Logic and Bit Operations/Compare To Constant  relop===  const=1  OutDataTypeStr=boolean
  Gain : Gain  Gain=10
  Relational Operator : RelationalOperator  Operator=<  OutDataTypeStr=boolean  RndMeth=Simplest
  tag scope: BW_Display=global
  wires:
  Compare To Constant5/1 -> [BW_Display]
  Inport/1 -> Compare To Constant/1
  Gain/1 -> Relational Operator/2
  Clock/1 -> Relational Operator/1
  Relational Operator/1 -> Compare To Constant5/1
  Compare To Constant/1 -> Gain/1

== system manual_model_features/MODULES/WIPER_CONTROL/Atomic Subsystem1 ==
  Inport : Inport
  Auto_Modes : Subsystem
  Display : Display
  Manual_mode : Subsystem
  wires:
  [FW_Modes] -> Manual_mode/1(In1), Auto_Modes/1(In1)
  Inport/1 -> Display/1
